simulink model "MyActiveSusp"  (R2021b)
settings: Solver=ode4  StartTime=0.0  StopTime=SIM_TIME  FixedStep=STEP_SIZE  RelTol=1e-3
undefined symbols (not defined in the file): b_s, b_t, k_s, k_t, m_s, m_u, x0
settings Model: Creator=tanzc  LastModifiedBy=tanzc
settings DataIOCC: ReturnWorkspaceOutputs=off

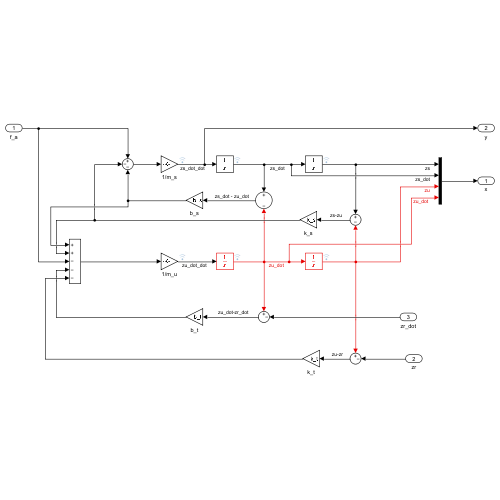
[thumbnail: Simulink's stored preview of the top-level diagram]
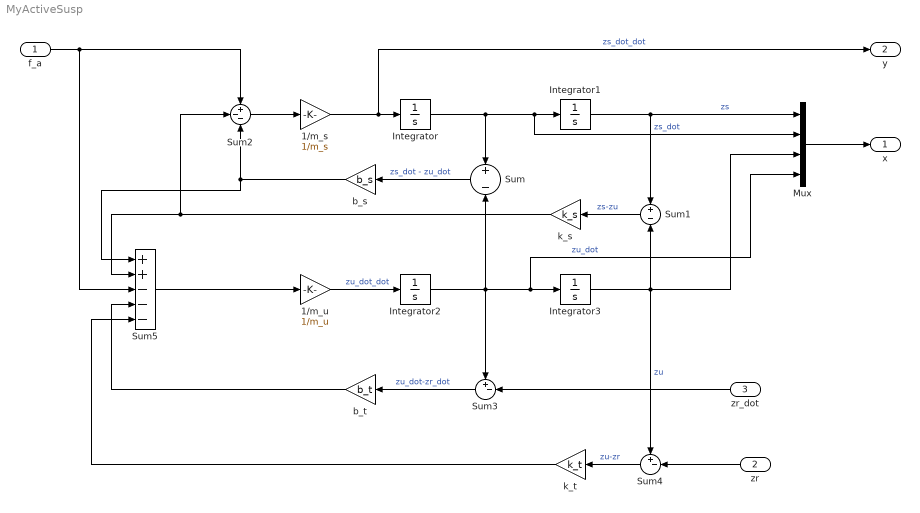
== system MyActiveSusp ==
  f_a : Inport
  zr : Inport  Port=2
  zr_dot : Inport  Port=3
  1/m_s : Gain  Gain=1/m_s
  1/m_u : Gain  Gain=1/m_u
  Integrator : Integrator
  Integrator1 : Integrator  InitialCondition=x0(1)
  Integrator2 : Integrator
  Integrator3 : Integrator
  Mux : Mux
  Sum : Sum  Inputs=+-
  Sum1 : Sum  Inputs=+-
  Sum2 : Sum  Inputs=+--
  Sum3 : Sum  Inputs=+-|
  Sum4 : Sum  Inputs=+-|
  Sum5 : Sum  Inputs=++---
  b_s : Gain  Gain=b_s
  b_t : Gain  Gain=b_t
  k_s : Gain  Gain=k_s
  k_t : Gain  Gain=k_t
  x : Outport
  y : Outport  Port=2
  wires:
  Integrator/1 -> Sum/1, Mux/2, Integrator1/1  "zs_dot"
  Sum2/1 -> 1/m_s/1
  Integrator1/1 -> Mux/1, Sum1/1  "zs"
  Integrator3/1 -> Mux/3, Sum4/1, Sum1/2  "zu"
  Sum5/1 -> 1/m_u/1
  Integrator2/1 -> Sum3/1, Sum/2, Mux/4, Integrator3/1  "zu_dot"
  Sum/1 -> b_s/1  "zs_dot - zu_dot"
  Sum1/1 -> k_s/1  "zs-zu"
  f_a/1 -> Sum5/3, Sum2/1
  b_s/1 -> Sum5/1, Sum2/3
  k_s/1 -> Sum5/2, Sum2/2
  1/m_s/1 -> y/1, Integrator/1  "zs_dot_dot"
  zr_dot/1 -> Sum3/2
  Sum3/1 -> b_t/1  "zu_dot-zr_dot"
  zr/1 -> Sum4/2
  Sum4/1 -> k_t/1  "zu-zr"
  b_t/1 -> Sum5/4
  k_t/1 -> Sum5/5
  1/m_u/1 -> Integrator2/1  "zu_dot_dot"
  Mux/1 -> x/1
